simulink model "surrogate_model_1"  (R2026a)
settings: Solver=VariableStepAuto
settings Model: Creator=shuki  LastModifiedBy=shuki

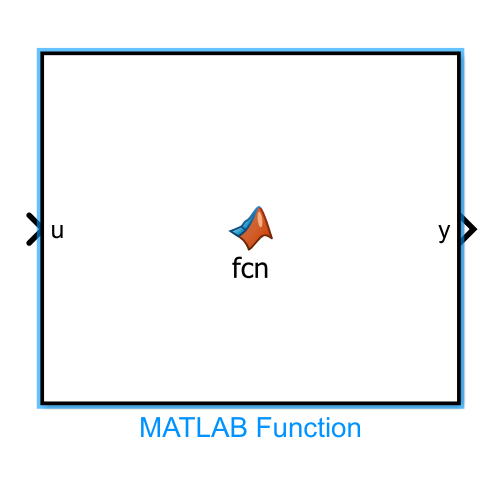
[thumbnail: Simulink's stored preview of the top-level diagram]
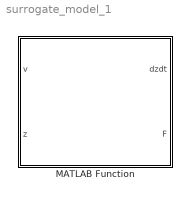
== system surrogate_model_1 ==
  MATLAB Function : MATLAB Function  TreatAsAtomicUnit=on

== matlab function surrogate_model_1/MATLAB Function ==
  data: v input; dzdt output; z input; F output
function [dzdt, F] = surrogate_model_1(v, z)

    C1 = 5.774465711;
    C2 = 0.70994425;
    
    dzdt = (v + z) - z * abs(C1 * (1e10 * z^2 - C2)^2 - 1e5 * abs(v + z));

    F = 1e5 * z + 316.2277 * dzdt + 0.4 * v;
end
